simulink model "third"  (Simulink 7.4)
settings: Solver=ode23tb  StartTime=0.0  StopTime=3  MaxStep=1e-5  RelTol=1e-3
undefined symbols (not defined in the file): powergui
libraries: powerlib x6, simulink x2, powerlib_extras x1
settings Model: Creator=lenovo  LastModifiedBy=lenovo
settings OptimizationCC: InitFltsAndDblsToZero=on
settings DebuggingCC: SaveWithParameterizedLinksMsg=none  SignalResolutionControl=TryResolveAllWithWarning  MultiTaskDSMMsg=warning  MultiTaskCondExecSysMsg=none
settings RTWCC: IncludeERTFirstTime=on
settings GRTTargetCC: TargetFcnLib=ansi_tfl_tmw.mat

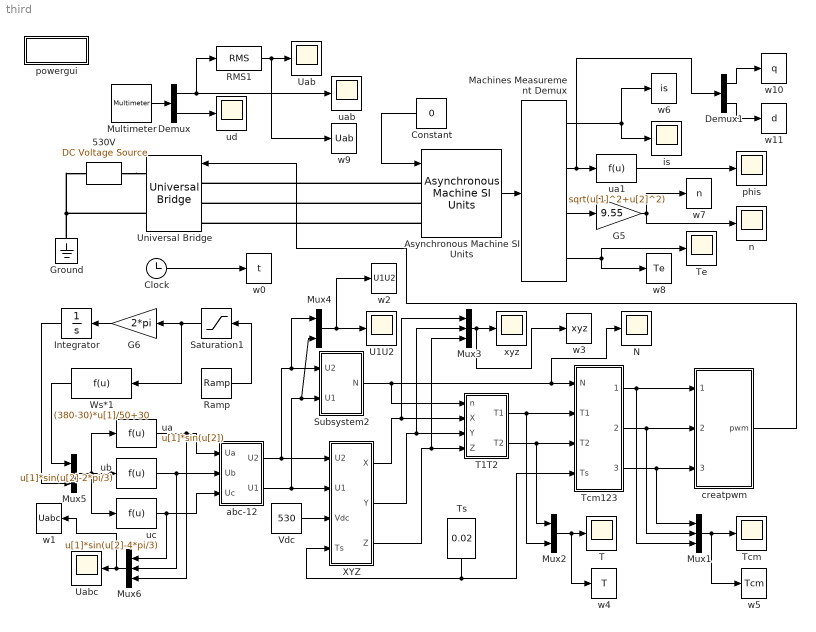
== system third ==
  530V : powerlib/Electrical Sources/DC Voltage Source  DialogController=POWERSYS.PowerSysDialog  SystemSampleTime=-1  Amplitude=530  Measurements=Voltage
  Asynchronous Machine SI Units : powerlib/Machines/Asynchronous Machine SI Units  DialogController=POWERSYS.PowerSysDialog  SystemSampleTime=-1  PresetModel=No  MechanicalLoad=Torque Tm  ShowDetailedParameters=on  RotorType=Squirrel-cage  ReferenceFrame=Rotor  NominalParameters=[2200 380 50]  Stator=[6.9 0.0455]  Rotor=[8.18 0.0455]  Lm=1.0039  Mechanical=[0.02 0.005752 2]  PolePairs=2  InitialConditions="[ 1,0   0,0,0   0,0,0 ]"  Units=SI  LoadFlowParameters=0  SimulateSaturation=off  Saturation=[9.9249,19.6672,38.0377,51.3988,69.2824,105.1337,152.5532,214.2421,303.1917;230, 322, 414, 460, 506, 552, 598, 644, 690]  TsPowergui=0  TsBlock=-1  IterativeModel=Forward Euler
  Clock : Clock
      settings: Decimation=10
  Constant : Constant  Value=0  OutDataType=sfix(16)  OutScaling=2^0
  Demux : Demux  Outputs=2
  Demux1 : Demux  Outputs=2
  G5 : Gain  Gain=9.55  ParameterDataType=sfix(16)  ParameterScaling=2^0  OutDataType=sfix(16)  OutScaling=2^0
  G6 : Gain  Gain=2*pi  ParameterDataType=sfix(16)  ParameterScaling=2^0  OutDataType=sfix(16)  OutScaling=2^0
  Ground : powerlib/Elements/Ground  DialogController=POWERSYS.PowerSysDialog  PhysicalDomain=powersysdomain  SubClassName=unknown  LeftPortType=p1  RightPortType=p1  LConnTagsString=a
  Integrator : Integrator
  Machines Measurement Demux : powerlib/Machines/Machines Measurement Demux  DialogController=POWERSYS.PowerSysDialog  SystemSampleTime=-1  machType=Asynchronous  ssm1=on  ssm2=on  ssm3=on  ssm4=on  ssm5=on  ssm6=on  sm1=off  sm2=off  sm3=off  sm4=off  sm5=off  sm6=off  sm7=off  sm8=on  sm9=off  sm10=off  sm11=off  sm115=off  sm12=off  sm13=off  sm14=off  asm1=off  asm2=off  asm3=off  asm4=off  asm5=on  asm6=off  asm7=on  asm8=off  asm9=on  asm10=on  asm11=off  pmsm1=on  pmsm2=on  pmsm3=on  pmsm4=off  pmsm5=on  pmsm6=on  pmsm7=on  lastType=1
  Multimeter : powerlib/Measurements/Multimeter  SystemSampleTime=-1  PhasorSimulation=off  OutputType=Complex  sel=[7 11]  L=17  Gain=[1 1]  yselected={'Uab: Universal Bridge','Usrc: 530V'};  PSBOutputType=1  PSBequivalent=0  AxesSetting=[0,0.1,-100,100]  Display=0  SavedBlockNames=-11
  Mux1 : Mux  Inputs=3
  Mux2 : Mux  Inputs=2
  Mux3 : Mux  Inputs=3
  Mux4 : Mux  Inputs=2
  Mux5 : Mux  Inputs=2
  Mux6 : Mux  Inputs=3
  N : Scope
      settings: YMin=0  YMax=1500  SaveName=T1  DataFormat=Array
  RMS1 : powerlib_extras/Measurements/RMS  DialogController=POWERSYS.PowerSysDialog  SystemSampleTime=-1  f1=60
  Ramp : simulink/Sources/Ramp  SystemSampleTime=-1  slope=50  start=0  X0=0
  Saturation1 : Saturate  UpperLimit=50
  Subsystem2 : Subsystem
  T : Scope
      settings: YMin=0  YMax=1500  SaveName=T  DataFormat=Array
  T1T2 : Subsystem
  Tcm : Scope
      settings: YMin=0.00225  YMax=0.00775  SaveName=Tcm  DataFormat=Array
  Tcm123 : Subsystem
  Te : Scope
      settings: YMin=0.9  YMax=2.4  SaveName=Te  DataFormat=Array
  Ts : Constant  Value=0.02  OutDataType=sfix(16)  OutScaling=2^0
  U1U2 : Scope
      settings: TimeRange=3  YMin=-125  YMax=150  SaveName=U1U2  DataFormat=Array
  Uab : Scope
      settings: YMin=147.5  YMax=177.5  SaveName=Uab  DataFormat=Array
  Uabc : Scope
      settings: YMin=-275  YMax=275  SaveName=Ua  DataFormat=Array
  Universal Bridge : powerlib/Power Electronics/Universal Bridge  DialogController=POWERSYS.PowerSysDialog  SystemSampleTime=-1  Arms=3  SnubberResistance=1e5  SnubberCapacitance=inf  Device=IGBT / Diodes  Ron=1e-3  Lon=0  ForwardVoltages="[  0  0  ]"  ForwardVoltage=0  GTOparameters=[ 10e-6 , 20e-6 ]  IGBTparameters=[ 1e-6 , 2e-6 ]  Measurements=All voltages and currents  Measurements_2=None  converterType=Rectifier
  Vdc : Constant  Value=530  OutDataType=sfix(16)  OutScaling=2^0
  Ws*1 : Fcn  Expr=(380-30)*u[1]/50+30
  XYZ : Subsystem
  abc-12 : Subsystem
  creatpwm : Subsystem
  is : Scope
      settings: YMin=-2  YMax=2  SaveName=is  DataFormat=Array
  n : Scope
      settings: YMin=1484.97  YMax=1485.05  SaveName=n  DataFormat=Array
  phis : Scope
      settings: YMin=-2  YMax=2  SaveName=is2  DataFormat=Array
  powergui : Subsystem  AncestorBlock=powerlib/powergui  InitFcn=powergui( 'InitFcn_Callback' , gcb , 0 , [ ] );  StopFcn=powergui( 'StopFcn_Callback' , gcb , 0 , [ ] );  mask(PSB option menu block){SimulationMode=Continuous, SampleTime=1e-5, frequency=60, SPID=off, DisableSnubberDevices=off, DisableRonSwitches=off, DisableVfSwitches=off, SwTol=0, Interpol=off, frequencyindice=50, echomessages=off, HookPort=off, DisplayEquations=off, FunctionMessages=off, EnableUseOfTLC=off, x0status=blocks, RestoreLinks=warning, Frange=[0:2:500], Ylog=off, Xlog=on, ShowGrid=off, save=off, variable=ZData, structure=, ZoomFFT=on, StartTime=0.0, cycles=1, DisplayStyle=1, fundamental=60, FreqAxis=off, MaxFrequency=1000, frequencyindicesteady=1, RmsSteady=1, display=off, Ts=0, methode=off}
      mask prompts: SimulationMode "Simulation type:"; SampleTime "Sample time (s):"; frequency "Phasor frequency (Hz):"; SPID "Enable use of ideal switching devices"; DisableSnubberDevices "Disable snubbers in switching devices"; DisableRonSwitches "Disable On resistance in switching devices (Ron=0)"; DisableVfSwitches "Disable Forward voltage in switching devices (Vf=0)"; SwTol "Switch tolerance"; Interpol "Interpolate"; frequencyindice "Load flow frequency (Hz):"; echomessages "Display SimPowerSystems warnings and messages"; HookPort "Add a hook port to the powergui block"; DisplayEquations "Display circuit differential equations"; FunctionMessages "Display internal function messages (debug mode feature)"; EnableUseOfTLC "Use TLC file when in Accelerator Simulation Mode and for RTW applications"; x0status "Start simulation with initial electrical states from:"; RestoreLinks "Restore disabled links of SimPowerSystems blocks:"; Frange "Frequency Range"; Ylog "Log impedance"; Xlog "log Frequency"; ShowGrid "grid"; save "Save Data To Workspace"; variable "Variable Name"; structure "Structure Name (PSBFFTSCOPE)"; ZoomFFT "ZoomFFT (PSBFFTSCOPE)"; StartTime "Start Time (PSBFFTSCOPE)"; cycles "Cycles (PSBFFTSCOPE)"; DisplayStyle "Display style (PSBFFTSCOPE)"; fundamental "Fundamental (PSBFFTSCOPE)"; FreqAxis "Frequency Axis (PSBFFTSCOPE)"; MaxFrequency "Max Frequency (PSBFFTSCOPE)"; frequencyindicesteady "Frequency indice (STEADYSTATE)"; RmsSteady "RMS display (STEADYSTATE)"; display "Display Results"; Ts "Old Ts setting (OBSOLETE)"; methode "Phasor simulation (OBSOLETE)"
      mask help: Set simulation type, simulation parameters, and preferences
      mask init:
      | message = powergui('MaskInitialization',gcb,SimulationMode,SampleTime);
      settings: CopyFcn=powergui( 'Copy_Callback' , gcb , 0 , [ ] );  ModelCloseFcn=powergui( 'CloseButton_Callback' , gcb , [ ] , [ ] );  NameChangeFcn=powergui( 'NameChangeFcn_Callback' , gcb , 0 , [ ] );  OpenFcn=powergui(gcb,'Open')
      settings: DeleteFcn=|
      | powergui( 'Copy_Callback' , gcb , 1 , [ ] );
      | powergui( 'CloseButton_Callback' , gcb , [ ] , [ ] );
      settings: PreSaveFcn=|
      | powergui( 'PreSaveFcn_Callback' , gcb , [ ] , [ ] );
      | powergui( 'CloseButton_Callback' , gcb , [ ] , [ ] );
      mask Help: web(psbhelp)
      mask StyleString: popup(Continuous|Discrete|Phasor),edit,edit,checkbox,checkbox,checkbox,checkbox,edit,checkbox,edit,checkbox,checkbox,checkbox,checkbox,checkbox,popup(blocks|steady|zero),popup(yes|warning|no),edit,checkbox,checkbox,checkbox,checkbox,edit,edit,checkbox,edit,edit,edit,edit,checkbox,edit,edit,edit,checkbox,edit,checkbox
      mask CallbackString: powergui('SimulationType',[],[],gcb);|||powergui('SPID',[],[],gcb);||||||||powergui('HookPort',[],[],gcb);||||||||||||||||||||||||
      mask TabNameString: Solver,Solver,Solver,Solver,Solver,Solver,Solver,Solver,Solver,Preferences,Preferences,Preferences,Solver,Solver,Preferences,Preferences,Preferences,Preferences,Preferences,Preferences,Preferences,Preferences,Preferences,Preferences,Preferences,Preferences,Preferences,Preferences,Preferences,Preferences,Preferences,Preferences,Preferences,Preferences,Solver,Solver
      mask Display: color('blue'),disp(message)
  ua : Fcn  Expr=u[1]*sin(u[2])
  ua1 : Fcn  Expr=sqrt(u[1]^2+u[2]^2)
  uab : Scope
      settings: YMin=0  YMax=1500  SaveName=uab  DataFormat=Array
  ub : Fcn  Expr=u[1]*sin(u[2]-2*pi/3)
  uc : Fcn  Expr=u[1]*sin(u[2]-4*pi/3)
  ud : Scope
      settings: YMin=0  YMax=1500  SaveName=ud  DataFormat=Array
  w0 : ToWorkspace  VariableName=t  SampleTime=-1  SaveFormat=Array
  w1 : ToWorkspace  VariableName=Uabc  SampleTime=-1  SaveFormat=Array
  w10 : ToWorkspace  VariableName=q  SampleTime=-1  SaveFormat=Array
  w11 : ToWorkspace  VariableName=d  SampleTime=-1  SaveFormat=Array
  w2 : ToWorkspace  VariableName=U1U2  SampleTime=-1  SaveFormat=Array
  w3 : ToWorkspace  VariableName=xyz  SampleTime=-1  SaveFormat=Array
  w4 : ToWorkspace  VariableName=T  SampleTime=-1  SaveFormat=Array
  w5 : ToWorkspace  VariableName=Tcm  SampleTime=-1  SaveFormat=Array
  w6 : ToWorkspace  VariableName=is  SampleTime=-1  SaveFormat=Array
  w7 : ToWorkspace  VariableName=n  SampleTime=-1  SaveFormat=Array
  w8 : ToWorkspace  VariableName=Te  SampleTime=-1  SaveFormat=Array
  w9 : ToWorkspace  VariableName=Uab  SampleTime=-1  SaveFormat=Array
  xyz : Scope
      settings: YMin=0  YMax=1500  SaveName=xyz  DataFormat=Array
  wires:
  Asynchronous Machine SI Units/1 -> Machines Measurement Demux/1
  Multimeter/1 -> Demux/1
  Demux/1 -> RMS1/1, uab/1
  Demux/2 -> ud/1
  Machines Measurement Demux/1 -> w6/1, is/1
  Machines Measurement Demux/3 -> G5/1
  G5/1 -> w7/1, n/1
  Machines Measurement Demux/4 -> Te/1, w8/1
  Constant/1 -> Asynchronous Machine SI Units/1
  Ramp/1 -> Saturation1/1
  G6/1 -> Integrator/1
  Ws*1/1 -> Mux5/1
  Integrator/1 -> Mux5/2
  Mux5/1 -> ub/1, ua/1, uc/1
  Ts/1 -> XYZ/4(Ts), Tcm123/4(Ts)
  Vdc/1 -> XYZ/3(Vdc)
  Subsystem2/1(N) -> T1T2/1(n), Tcm123/1(N), N/1
  XYZ/1(X) -> T1T2/2(X), Mux3/1
  XYZ/2(Y) -> T1T2/3(Y), Mux3/2
  XYZ/3(Z) -> T1T2/4(Z), Mux3/3
  T1T2/1(T1) -> Tcm123/2(T1), Mux2/2
  T1T2/2(T2) -> Tcm123/3(T2), Mux2/1
  Tcm123/1(Tcm1) -> creatpwm/1(Tcm1), Mux1/3
  Tcm123/2(Tcm2) -> creatpwm/2(Tcm2), Mux1/2
  Tcm123/3(Tcm3) -> creatpwm/3(Tcm3), Mux1/1
  ua/1 -> abc-12/1(Ua), Mux6/3
  ub/1 -> abc-12/2(Ub), Mux6/2
  uc/1 -> abc-12/3(Uc), Mux6/1
  RMS1/1 -> Uab/1, w9/1
  abc-12/1(U2) -> XYZ/1(U2), Subsystem2/1(U2), Mux4/1
  abc-12/2(U1) -> XYZ/2(U1), Subsystem2/2(U1), Mux4/2
  Saturation1/1 -> G6/1, Ws*1/1
  Mux1/1 -> Tcm/1, w5/1
  Mux2/1 -> T/1, w4/1
  Mux3/1 -> w3/1, xyz/1
  Mux4/1 -> U1U2/1, w2/1
  Mux6/1 -> Uabc/1, w1/1
  Clock/1 -> w0/1
  ua1/1 -> phis/1
  creatpwm/1(pwm) -> Universal Bridge/1
  Machines Measurement Demux/2 -> ua1/1, Demux1/1
  Demux1/1 -> w10/1
  Demux1/2 -> w11/1
  connections:
  Asynchronous Machine SI Units/LConn1 -- Universal Bridge/LConn1
  Asynchronous Machine SI Units/LConn2 -- Universal Bridge/LConn2
  Asynchronous Machine SI Units/LConn3 -- Universal Bridge/LConn3
  Ground/LConn1 -- 530V/LConn1 -- Universal Bridge/RConn2
  530V/RConn1 -- Universal Bridge/RConn1

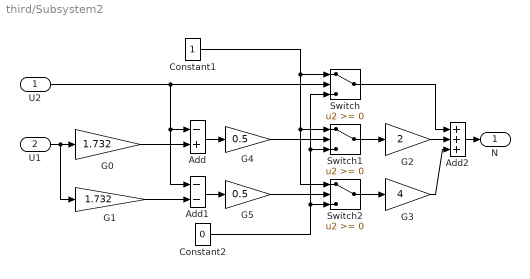
== system third/Subsystem2 ==
  U2 : Inport  OutDataType=sfix(16)  OutScaling=2^0
  U1 : Inport  Port=2  OutDataType=sfix(16)  OutScaling=2^0
  Add : Sum  Inputs=-+  OutDataType=sfix(16)  OutScaling=2^-10
  Add1 : Sum  Inputs=--  OutDataType=sfix(16)  OutScaling=2^-10
  Add2 : Sum  Inputs=+++  OutDataType=sfix(16)  OutScaling=2^-10
  Constant1 : Constant  OutDataType=sfix(16)  OutScaling=2^0
  Constant2 : Constant  Value=0  OutDataType=sfix(16)  OutScaling=2^0
  G0 : Gain  Gain=1.732  ParameterDataType=sfix(16)  ParameterScaling=2^0  OutDataType=sfix(16)  OutScaling=2^0
  G1 : Gain  Gain=1.732  ParameterDataType=sfix(16)  ParameterScaling=2^0  OutDataType=sfix(16)  OutScaling=2^0
  G2 : Gain  Gain=2  ParameterDataType=sfix(16)  ParameterScaling=2^0  OutDataType=sfix(16)  OutScaling=2^0
  G3 : Gain  Gain=4  ParameterDataType=sfix(16)  ParameterScaling=2^0  OutDataType=sfix(16)  OutScaling=2^0
  G4 : Gain  Gain=0.5  ParameterDataType=sfix(16)  ParameterScaling=2^0  OutDataType=sfix(16)  OutScaling=2^0
  G5 : Gain  Gain=0.5  ParameterDataType=sfix(16)  ParameterScaling=2^0  OutDataType=sfix(16)  OutScaling=2^0
  Switch : Switch
  Switch1 : Switch
  Switch2 : Switch
  N : Outport  OutDataType=sfix(16)  OutScaling=2^0
  wires:
  Add2/1 -> N/1
  Switch/1 -> Add2/1
  G3/1 -> Add2/3
  G2/1 -> Add2/2
  Switch1/1 -> G2/1
  Switch2/1 -> G3/1
  Add1/1 -> G5/1
  Constant2/1 -> Switch2/3, Switch1/3, Switch/3
  Add/1 -> G4/1
  Constant1/1 -> Switch2/1, Switch1/1, Switch/1
  U2/1 -> Add1/1, Add/1, Switch/2
  G1/1 -> Add1/2
  U1/1 -> G1/1, G0/1
  G0/1 -> Add/2
  G4/1 -> Switch1/2
  G5/1 -> Switch2/2

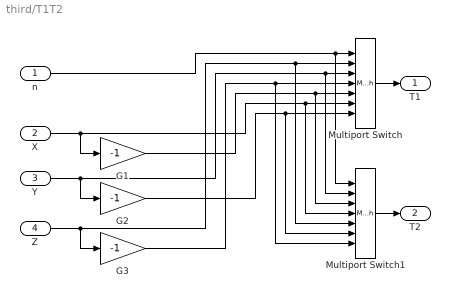
== system third/T1T2 ==
  n : Inport  OutDataType=sfix(16)  OutScaling=2^0
  X : Inport  Port=2  OutDataType=sfix(16)  OutScaling=2^0
  Y : Inport  Port=3  OutDataType=sfix(16)  OutScaling=2^0
  Z : Inport  Port=4  OutDataType=sfix(16)  OutScaling=2^0
  G1 : Gain  Gain=-1  ParameterDataType=sfix(16)  ParameterScaling=2^0  OutDataType=sfix(16)  OutScaling=2^0
  G2 : Gain  Gain=-1  ParameterDataType=sfix(16)  ParameterScaling=2^0  OutDataType=sfix(16)  OutScaling=2^0
  G3 : Gain  Gain=-1  ParameterDataType=sfix(16)  ParameterScaling=2^0  OutDataType=sfix(16)  OutScaling=2^0
  Multiport Switch : MultiPortSwitch  Inputs=6
  Multiport Switch1 : MultiPortSwitch  Inputs=6
  T1 : Outport  OutDataType=sfix(16)  OutScaling=2^0
  T2 : Outport  Port=2  OutDataType=sfix(16)  OutScaling=2^0
  wires:
  G2/1 -> Multiport Switch1/6, Multiport Switch/7
  G3/1 -> Multiport Switch1/7, Multiport Switch/4
  G1/1 -> Multiport Switch1/3, Multiport Switch/5
  Z/1 -> Multiport Switch1/5, Multiport Switch/2, G3/1
  Y/1 -> Multiport Switch1/2, Multiport Switch/3, G2/1
  X/1 -> Multiport Switch1/4, Multiport Switch/6, G1/1
  n/1 -> Multiport Switch1/1, Multiport Switch/1
  Multiport Switch1/1 -> T2/1
  Multiport Switch/1 -> T1/1

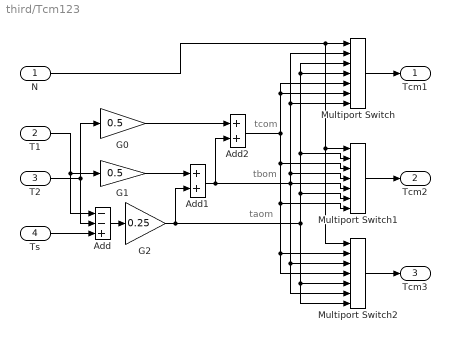
== system third/Tcm123 ==
  note: taom
  note: tbom
  note: tcom
  N : Inport  OutDataType=sfix(16)  OutScaling=2^0
  T1 : Inport  Port=2  OutDataType=sfix(16)  OutScaling=2^0
  T2 : Inport  Port=3  OutDataType=sfix(16)  OutScaling=2^0
  Ts : Inport  Port=4  OutDataType=sfix(16)  OutScaling=2^0
  Add : Sum  Inputs=--+  OutDataType=sfix(16)  OutScaling=2^-10
  Add1 : Sum  OutDataType=sfix(16)  OutScaling=2^-10
  Add2 : Sum  OutDataType=sfix(16)  OutScaling=2^-10
  G0 : Gain  Gain=0.5  ParameterDataType=sfix(16)  ParameterScaling=2^0  OutDataType=sfix(16)  OutScaling=2^0
  G1 : Gain  Gain=0.5  ParameterDataType=sfix(16)  ParameterScaling=2^0  OutDataType=sfix(16)  OutScaling=2^0
  G2 : Gain  Gain=0.25  ParameterDataType=sfix(16)  ParameterScaling=2^0  OutDataType=sfix(16)  OutScaling=2^0
  Multiport Switch : MultiPortSwitch  Inputs=6
  Multiport Switch1 : MultiPortSwitch  Inputs=6
  Multiport Switch2 : MultiPortSwitch  Inputs=6
  Tcm1 : Outport  OutDataType=sfix(16)  OutScaling=2^0
  Tcm2 : Outport  Port=2  OutDataType=sfix(16)  OutScaling=2^0
  Tcm3 : Outport  Port=3  OutDataType=sfix(16)  OutScaling=2^0
  wires:
  Add2/1 -> Multiport Switch1/3, Multiport Switch2/4, Multiport Switch2/2, Multiport Switch1/7, Multiport Switch/5, Multiport Switch/6
  Add1/1 -> Multiport Switch2/6, Multiport Switch2/3, Multiport Switch1/5, Multiport Switch1/4, Multiport Switch/2, Multiport Switch/7, Add2/2
  G2/1 -> Multiport Switch2/5, Multiport Switch2/7, Multiport Switch1/6, Multiport Switch1/2, Multiport Switch/4, Multiport Switch/3, Add1/2
  G1/1 -> Add1/1
  G0/1 -> Add2/1
  Add/1 -> G2/1
  Ts/1 -> Add/3
  T2/1 -> Add/2, G0/1
  T1/1 -> Add/1, G1/1
  Multiport Switch2/1 -> Tcm3/1
  Multiport Switch1/1 -> Tcm2/1
  N/1 -> Multiport Switch/1, Multiport Switch2/1, Multiport Switch1/1
  Multiport Switch/1 -> Tcm1/1

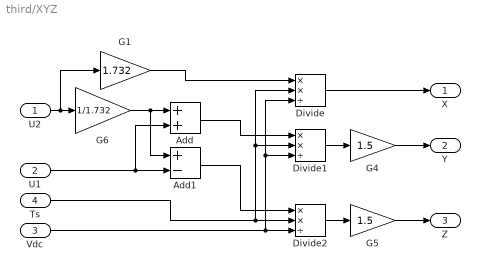
== system third/XYZ ==
  U2 : Inport  OutDataType=sfix(16)  OutScaling=2^0
  U1 : Inport  Port=2  OutDataType=sfix(16)  OutScaling=2^0
  Vdc : Inport  Port=3  OutDataType=sfix(16)  OutScaling=2^0
  Ts : Inport  Port=4  OutDataType=sfix(16)  OutScaling=2^0
  Add : Sum  OutDataType=sfix(16)  OutScaling=2^-10
  Add1 : Sum  Inputs=+-  OutDataType=sfix(16)  OutScaling=2^-10
  Divide : Product  Inputs=**/  OutDataType=sfix(16)  OutScaling=2^-10
  Divide1 : Product  Inputs=**/  OutDataType=sfix(16)  OutScaling=2^-10
  Divide2 : Product  Inputs=**/  OutDataType=sfix(16)  OutScaling=2^-10
  G1 : Gain  Gain=1.732  ParameterDataType=sfix(16)  ParameterScaling=2^0  OutDataType=sfix(16)  OutScaling=2^0
  G4 : Gain  Gain=1.5  ParameterDataType=sfix(16)  ParameterScaling=2^0  OutDataType=sfix(16)  OutScaling=2^0
  G5 : Gain  Gain=1.5  ParameterDataType=sfix(16)  ParameterScaling=2^0  OutDataType=sfix(16)  OutScaling=2^0
  G6 : Gain  Gain=1/1.732  ParameterDataType=sfix(16)  ParameterScaling=2^0  OutDataType=sfix(16)  OutScaling=2^0
  X : Outport  OutDataType=sfix(16)  OutScaling=2^0
  Y : Outport  Port=2  OutDataType=sfix(16)  OutScaling=2^0
  Z : Outport  Port=3  OutDataType=sfix(16)  OutScaling=2^0
  wires:
  Divide/1 -> X/1
  G4/1 -> Y/1
  G5/1 -> Z/1
  Divide2/1 -> G5/1
  Divide1/1 -> G4/1
  Vdc/1 -> Divide/3, Divide1/3, Divide2/3
  Ts/1 -> Divide/2, Divide1/2, Divide2/2
  Add1/1 -> Divide2/1
  Add/1 -> Divide1/1
  G1/1 -> Divide/1
  U1/1 -> Add1/2, Add/2
  U2/1 -> G1/1, G6/1
  G6/1 -> Add/1, Add1/1

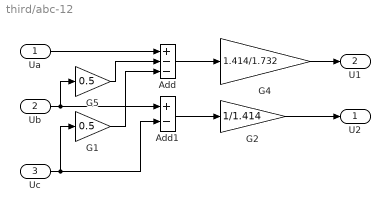
== system third/abc-12 ==
  Ua : Inport  OutDataType=sfix(16)  OutScaling=2^0
  Ub : Inport  Port=2  OutDataType=sfix(16)  OutScaling=2^0
  Uc : Inport  Port=3  OutDataType=sfix(16)  OutScaling=2^0
  Add : Sum  Inputs=+--  OutDataType=sfix(16)  OutScaling=2^-10
  Add1 : Sum  Inputs=+-  OutDataType=sfix(16)  OutScaling=2^-10
  G1 : Gain  Gain=0.5  ParameterDataType=sfix(16)  ParameterScaling=2^0  OutDataType=sfix(16)  OutScaling=2^0
  G2 : Gain  Gain=1/1.414  ParameterDataType=sfix(16)  ParameterScaling=2^0  OutDataType=sfix(16)  OutScaling=2^0
  G4 : Gain  Gain=1.414/1.732  ParameterDataType=sfix(16)  ParameterScaling=2^0  OutDataType=sfix(16)  OutScaling=2^0
  G5 : Gain  Gain=0.5  ParameterDataType=sfix(16)  ParameterScaling=2^0  OutDataType=sfix(16)  OutScaling=2^0
  U2 : Outport  OutDataType=sfix(16)  OutScaling=2^0
  U1 : Outport  Port=2  OutDataType=sfix(16)  OutScaling=2^0
  wires:
  Ua/1 -> Add/1
  Ub/1 -> G5/1, Add1/1
  G2/1 -> U2/1
  Uc/1 -> G1/1, Add1/2
  Add/1 -> G4/1
  G4/1 -> U1/1
  Add1/1 -> G2/1
  G5/1 -> Add/2
  G1/1 -> Add/3

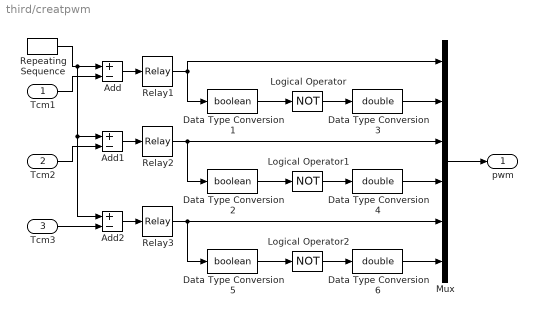
== system third/creatpwm ==
  Tcm1 : Inport  OutDataType=sfix(16)  OutScaling=2^0
  Tcm2 : Inport  Port=2  OutDataType=sfix(16)  OutScaling=2^0
  Tcm3 : Inport  Port=3  OutDataType=sfix(16)  OutScaling=2^0
  Add : Sum  Inputs=+-  OutDataType=sfix(16)  OutScaling=2^-10
  Add1 : Sum  Inputs=+-  OutDataType=sfix(16)  OutScaling=2^-10
  Add2 : Sum  Inputs=+-  OutDataType=sfix(16)  OutScaling=2^-10
  Data Type Conversion1 : DataTypeConversion  OutDataTypeMode=boolean  OutDataType=sfix(16)  OutScaling=2^0  OutDataTypeStr=boolean
  Data Type Conversion2 : DataTypeConversion  OutDataTypeMode=boolean  OutDataType=sfix(16)  OutScaling=2^0  OutDataTypeStr=boolean
  Data Type Conversion3 : DataTypeConversion  OutDataTypeMode=double  OutDataType=sfix(16)  OutScaling=2^0  OutDataTypeStr=double
  Data Type Conversion4 : DataTypeConversion  OutDataTypeMode=double  OutDataType=sfix(16)  OutScaling=2^0  OutDataTypeStr=double
  Data Type Conversion5 : DataTypeConversion  OutDataTypeMode=boolean  OutDataType=sfix(16)  OutScaling=2^0  OutDataTypeStr=boolean
  Data Type Conversion6 : DataTypeConversion  OutDataTypeMode=double  OutDataType=sfix(16)  OutScaling=2^0  OutDataTypeStr=double
  Logical Operator : Logic  Operator=NOT  AllPortsSameDT=off  OutDataTypeMode=boolean  OutDataTypeStr=boolean
  Logical Operator1 : Logic  Operator=NOT  AllPortsSameDT=off  OutDataTypeMode=boolean  OutDataTypeStr=boolean
  Logical Operator2 : Logic  Operator=NOT  AllPortsSameDT=off  OutDataTypeMode=boolean  OutDataTypeStr=boolean
  Mux : Mux  Inputs=6
  Relay1 : Relay  OutDataType=sfix(16)  OutScaling=2^0
  Relay2 : Relay  OutDataType=sfix(16)  OutScaling=2^0
  Relay3 : Relay  OutDataType=sfix(16)  OutScaling=2^0
  Repeating Sequence : simulink/Sources/Repeating Sequence  SystemSampleTime=-1  rep_seq_t=[0 5e-4]  rep_seq_y=[-0.003 0.013]
  pwm : Outport  OutDataType=sfix(16)  OutScaling=2^0
  wires:
  Mux/1 -> pwm/1
  Tcm1/1 -> Add/2
  Logical Operator2/1 -> Data Type Conversion6/1
  Data Type Conversion5/1 -> Logical Operator2/1
  Logical Operator1/1 -> Data Type Conversion4/1
  Data Type Conversion2/1 -> Logical Operator1/1
  Logical Operator/1 -> Data Type Conversion3/1
  Data Type Conversion1/1 -> Logical Operator/1
  Relay1/1 -> Mux/1, Data Type Conversion1/1
  Relay3/1 -> Mux/5, Data Type Conversion5/1
  Relay2/1 -> Mux/3, Data Type Conversion2/1
  Add2/1 -> Relay3/1
  Add1/1 -> Relay2/1
  Add/1 -> Relay1/1
  Tcm3/1 -> Add2/2
  Tcm2/1 -> Add1/2
  Data Type Conversion3/1 -> Mux/2
  Data Type Conversion4/1 -> Mux/4
  Data Type Conversion6/1 -> Mux/6
  Repeating Sequence/1 -> Add/1, Add1/1, Add2/1

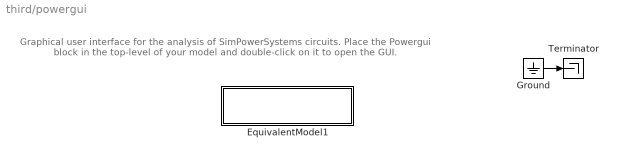
== system third/powergui ==
  note: Graphical user interface for the analysis of  SimPowerSystems circuits.
      | Place the Powergui block in the top-level of your model and double-click
      | on it to open the GUI.
  EquivalentModel1 : Subsystem
      mask init:
      | S  = GetDataForEquivalentModel('Continuous',gcbh);
      mask Display:
      | color('blue')
      | disp('EQUIVALENT CIRCUIT\nContinuous')
  Ground : Ground
  Terminator : Terminator
  wires:
  Ground/1 -> Terminator/1

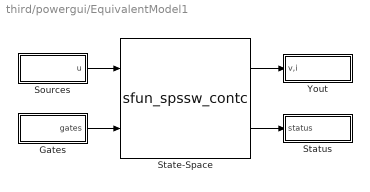
== system third/powergui/EquivalentModel1 ==
  Gates : Subsystem
  Sources : Subsystem
  State-Space : S-Function  FunctionName=sfun_spssw_contc  Parameters=S.A, S.B, S.C, S.D, S.x0, S.EnableUseOfTLC,S.SwitchResistance ,S.SwitchType, S.SwitchGateInitialValue, S.OutputsToResetToZero  EnableBusSupport=off
  Status : Subsystem
  Yout : Subsystem
  wires:
  State-Space/1 -> Yout/1(v,i)
  State-Space/2 -> Status/1(status)
  Sources/1(u) -> State-Space/1
  Gates/1(gates) -> State-Space/2

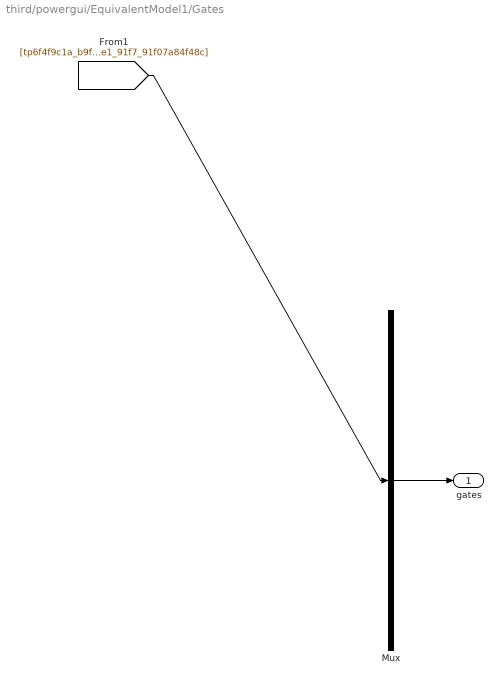
== system third/powergui/EquivalentModel1/Gates ==
  Mux : Mux  Inputs=1
  gates : Outport  OutDataType=sfix(16)  OutScaling=2^0
  wires:
  Mux/1 -> gates/1
  [tp6f4f9c1a_b9fe_48e1_91f7_91f07a84f48c] -> Mux/1

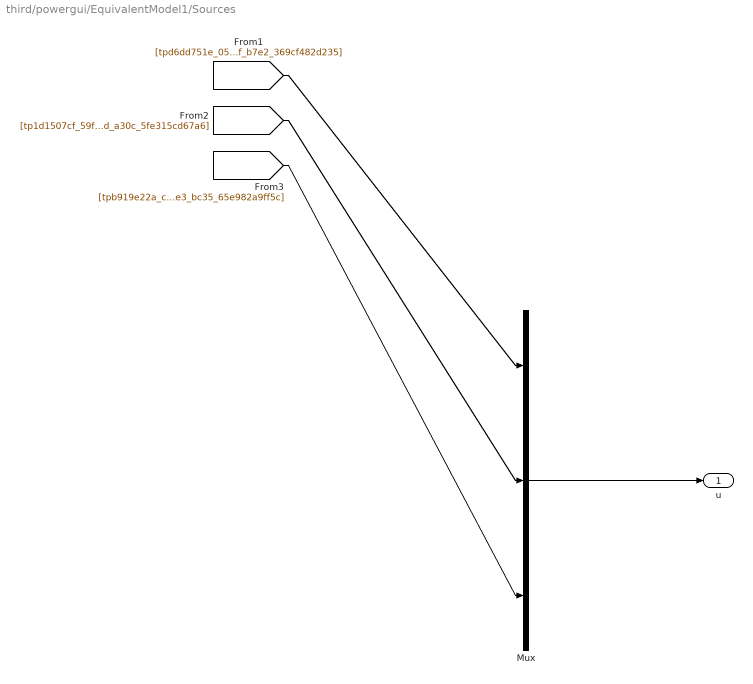
== system third/powergui/EquivalentModel1/Sources ==
  Mux : Mux  Inputs=[6 2 1]
  u : Outport  OutDataType=sfix(16)  OutScaling=2^0
  wires:
  Mux/1 -> u/1
  [tpd6dd751e_0511_495f_b7e2_369cf482d235] -> Mux/1
  [tp1d1507cf_59fa_4bad_a30c_5fe315cd67a6] -> Mux/2
  [tpb919e22a_cdf5_47e3_bc35_65e982a9ff5c] -> Mux/3

== system third/powergui/EquivalentModel1/Status ==
  status : Inport  OutDataType=sfix(16)  OutScaling=2^0
  Demux : Demux  Outputs=1
  tag scope: tpad003c7e_90e3_454f_aa40_739281f1c635=global
  wires:
  status/1 -> Demux/1
  Demux/1 -> [tpad003c7e_90e3_454f_aa40_739281f1c635]

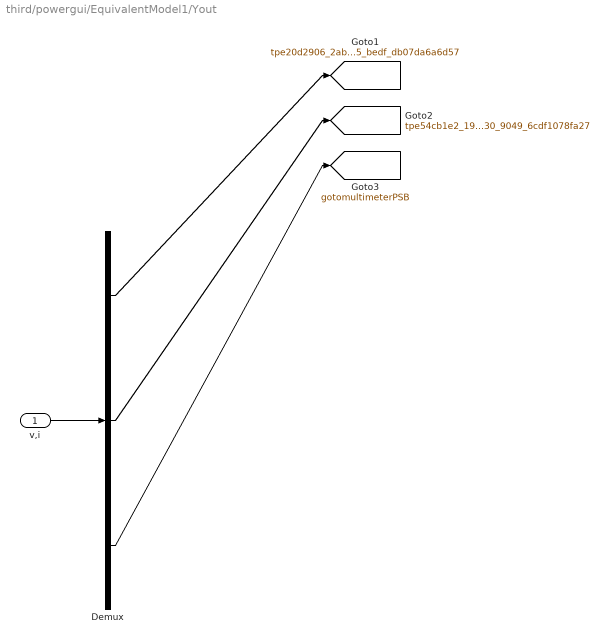
== system third/powergui/EquivalentModel1/Yout ==
  v,i : Inport  OutDataType=sfix(16)  OutScaling=2^0
  Demux : Demux  Outputs=[6 2 17]
  tag scope: gotomultimeterPSB=global, tpe20d2906_2ab0_45e5_bedf_db07da6a6d57=global, tpe54cb1e2_190a_4030_9049_6cdf1078fa27=global
  wires:
  v,i/1 -> Demux/1
  Demux/1 -> [tpe20d2906_2ab0_45e5_bedf_db07da6a6d57]
  Demux/2 -> [tpe54cb1e2_190a_4030_9049_6cdf1078fa27]
  Demux/3 -> [gotomultimeterPSB]
